simulink model "Defrost_3"  (R2022b)
settings: Solver=VariableStepAuto  StartTime=0.0  StopTime=100.0  RelTol=1e-3
InitFcn:
  | SNA = 170.5;
  | Temp_am = 4.5;
  | Tdef = 10;
  | Tdef_Second = 5;
  | Tbatt1 = 1;
  | Tbatt2 = 1;
  | RearDef_Voltage_L = 11.5;
  | RearDef_Voltage_H = 12;
undefined symbols (not defined in the file): sigbuilder_block
libraries: simulink x8
settings Model: Creator=muham  LastModifiedBy=muham

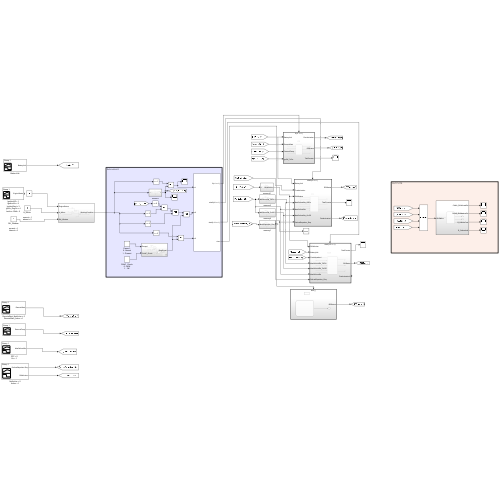
[thumbnail: Simulink's stored preview of the top-level diagram]
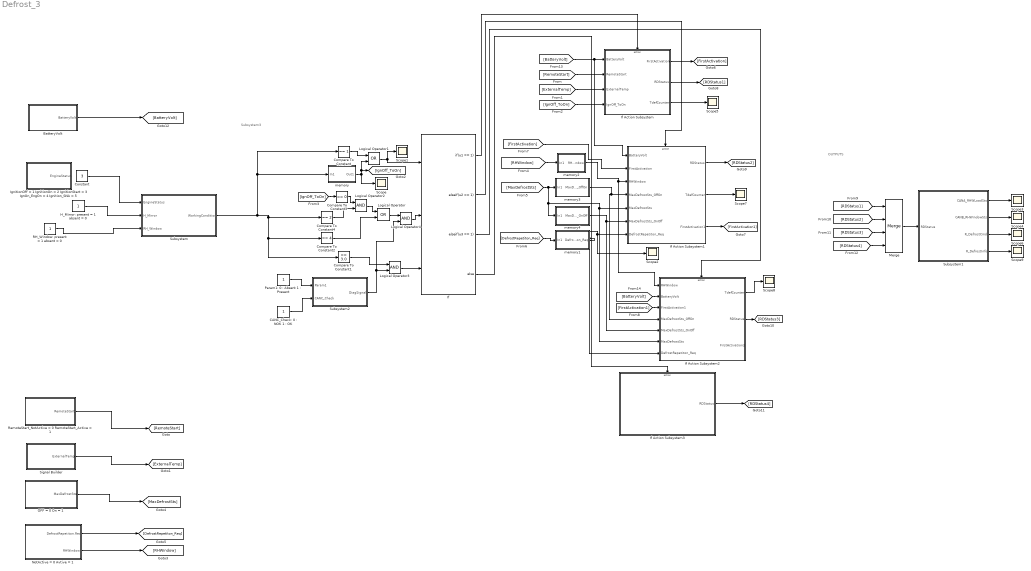
== system Defrost_3 ==
  note: Subsystem3
  note: OUTPUTS
  BatteryVolt : Subsystem  Tag=STV Subsys  LoadFcn=sigbuilder_block('load');  StartFcn=sigbuilder_block('start');  StopFcn=sigbuilder_block('stop');  ClipboardFcn=sigbuilder_block('clipboard');  mask(Sigbuilder block){tuvar=[0:10]}
      mask help: Simulink:masks:SigbuilderBlock_MD
      mask init:
      | if ~strcmp(get_param(bdroot(gcbh),'SimulationStatus'),'stopped') tuvar = sigbuilder_block('maskInit'); end
      settings: CopyFcn=sigbuilder_block('copy');  DeleteFcn=sigbuilder_block('delete');  ModelCloseFcn=sigbuilder_block('modelClose');  PreSaveFcn=sigbuilder_block('preSave');  PauseFcn=sigbuilder_block('pause');  ContinueFcn=sigbuilder_block('continue');  NameChangeFcn=sigbuilder_block('namechange');  OpenFcn=sigbuilder_block('open',[404.625 118.125 550.5 364.5 ]);  CloseFcn=sigbuilder_block('close');
      mask Display: plot(0, 0, 100, 100,[2, 2, 32, 32, 2], [68, 8, 8, 68, 68],[32, 2], [38, 38], [32, 19, 2],[53, 60, 44], [32, 17, 17, 2],[16, 16, 31, 31]);txt = getActiveGroup(gcbh);text(2, 100, txt,'verticalAlignment', 'top');
  "CANC_Check: 0 : NOK 1 : OK" : Constant
  Compare To Constant : simulink/Logic and Bit Operations/Compare To Constant  relop===  const=1  OutDataTypeStr=boolean
  Compare To Constant1 : simulink/Logic and Bit Operations/Compare To Constant  relop===  const=3.0  OutDataTypeStr=boolean
  Compare To Constant2 : simulink/Logic and Bit Operations/Compare To Constant  relop===  const=4  OutDataTypeStr=boolean
  Compare To Constant3 : simulink/Logic and Bit Operations/Compare To Constant  relop===  const=0  OutDataTypeStr=boolean
  Compare To Constant4 : simulink/Logic and Bit Operations/Compare To Constant  relop===  const=2  OutDataTypeStr=boolean
  Constant : Constant  Value=3
  H_Mirror: present = 1 absent = 0 : Constant
  If : If  NumInputs=3  IfExpression=u1 == 1  ElseIfExpressions=u2 == 1, u3 == 1
  If Action Subsystem : Subsystem  TreatAsAtomicUnit=on
  If Action Subsystem1 : Subsystem  TreatAsAtomicUnit=on
  If Action Subsystem2 : Subsystem  TreatAsAtomicUnit=on
  If Action Subsystem3 : Subsystem  TreatAsAtomicUnit=on
  IgnitionOff = 1 IgnitionOn = 2 IgnitionStart = 3 IgnOn_EngOn = 4 Ignition_SNA = 5 : Subsystem  Tag=STV Subsys  LoadFcn=sigbuilder_block('load');  StartFcn=sigbuilder_block('start');  StopFcn=sigbuilder_block('stop');  ClipboardFcn=sigbuilder_block('clipboard');  mask(Sigbuilder block){tuvar=[0:10]}
      mask help: Simulink:masks:SigbuilderBlock_MD
      mask init:
      | if ~strcmp(get_param(bdroot(gcbh),'SimulationStatus'),'stopped') tuvar = sigbuilder_block('maskInit'); end
      settings: CopyFcn=sigbuilder_block('copy');  DeleteFcn=sigbuilder_block('delete');  ModelCloseFcn=sigbuilder_block('modelClose');  PreSaveFcn=sigbuilder_block('preSave');  PauseFcn=sigbuilder_block('pause');  ContinueFcn=sigbuilder_block('continue');  NameChangeFcn=sigbuilder_block('namechange');  OpenFcn=sigbuilder_block('open',[73.125 79.125 550.5 364.5 ]);  CloseFcn=sigbuilder_block('close');
      mask Display: plot(0, 0, 100, 100,[2, 2, 32, 32, 2], [68, 8, 8, 68, 68],[32, 2], [38, 38], [32, 19, 2],[53, 60, 44], [32, 17, 17, 2],[16, 16, 31, 31]);txt = getActiveGroup(gcbh);text(2, 100, txt,'verticalAlignment', 'top');
  Logical Operator : Logic  Operator=OR  AllPortsSameDT=off  OutDataTypeStr=boolean
  Logical Operator1 : Logic  Operator=OR  AllPortsSameDT=off  OutDataTypeStr=boolean
  Logical Operator2 : Logic  AllPortsSameDT=off  OutDataTypeStr=boolean
  Logical Operator3 : Logic  AllPortsSameDT=off  OutDataTypeStr=boolean
  Logical Operator4 : Logic  AllPortsSameDT=off  OutDataTypeStr=boolean
  Merge : Merge  Inputs=4
  NotActive = 0 Avtive = 1 : Subsystem  Tag=STV Subsys  LoadFcn=sigbuilder_block('load');  StartFcn=sigbuilder_block('start');  StopFcn=sigbuilder_block('stop');  ClipboardFcn=sigbuilder_block('clipboard');  mask(Sigbuilder block){tuvar=[0:10]}
      mask help: Simulink:masks:SigbuilderBlock_MD
      mask init:
      | if ~strcmp(get_param(bdroot(gcbh),'SimulationStatus'),'stopped') tuvar = sigbuilder_block('maskInit'); end
      settings: CopyFcn=sigbuilder_block('copy');  DeleteFcn=sigbuilder_block('delete');  ModelCloseFcn=sigbuilder_block('modelClose');  PreSaveFcn=sigbuilder_block('preSave');  PauseFcn=sigbuilder_block('pause');  ContinueFcn=sigbuilder_block('continue');  NameChangeFcn=sigbuilder_block('namechange');  OpenFcn=sigbuilder_block('open',[404.625 118.125 550.5 364.5 ]);  CloseFcn=sigbuilder_block('close');
      mask Display: plot(0, 0, 100, 100,[2, 2, 32, 32, 2], [68, 8, 8, 68, 68],[32, 2], [38, 38], [32, 19, 2],[53, 60, 44], [32, 17, 17, 2],[16, 16, 31, 31]);txt = getActiveGroup(gcbh);text(2, 100, txt,'verticalAlignment', 'top');
  OFF = 0 On = 1 : Subsystem  Tag=STV Subsys  LoadFcn=sigbuilder_block('load');  StartFcn=sigbuilder_block('start');  StopFcn=sigbuilder_block('stop');  ClipboardFcn=sigbuilder_block('clipboard');  mask(Sigbuilder block){tuvar=[0:10]}
      mask help: Simulink:masks:SigbuilderBlock_MD
      mask init:
      | if ~strcmp(get_param(bdroot(gcbh),'SimulationStatus'),'stopped') tuvar = sigbuilder_block('maskInit'); end
      settings: CopyFcn=sigbuilder_block('copy');  DeleteFcn=sigbuilder_block('delete');  ModelCloseFcn=sigbuilder_block('modelClose');  PreSaveFcn=sigbuilder_block('preSave');  PauseFcn=sigbuilder_block('pause');  ContinueFcn=sigbuilder_block('continue');  NameChangeFcn=sigbuilder_block('namechange');  OpenFcn=sigbuilder_block('open',[404.625 118.125 550.5 364.5 ]);  CloseFcn=sigbuilder_block('close');
      mask Display: plot(0, 0, 100, 100,[2, 2, 32, 32, 2], [68, 8, 8, 68, 68],[32, 2], [38, 38], [32, 19, 2],[53, 60, 44], [32, 17, 17, 2],[16, 16, 31, 31]);txt = getActiveGroup(gcbh);text(2, 100, txt,'verticalAlignment', 'top');
  "Param1: 0 : Absent 1 : Present" : Constant
  RH_Window: present = 1 absent = 0 : Constant
  RemoteStart_NotActive = 0 RemoteStart_Active = 1 : Subsystem  Tag=STV Subsys  LoadFcn=sigbuilder_block('load');  StartFcn=sigbuilder_block('start');  StopFcn=sigbuilder_block('stop');  ClipboardFcn=sigbuilder_block('clipboard');  mask(Sigbuilder block){tuvar=[0:10]}
      mask help: Simulink:masks:SigbuilderBlock_MD
      mask init:
      | if ~strcmp(get_param(bdroot(gcbh),'SimulationStatus'),'stopped') tuvar = sigbuilder_block('maskInit'); end
      settings: CopyFcn=sigbuilder_block('copy');  DeleteFcn=sigbuilder_block('delete');  ModelCloseFcn=sigbuilder_block('modelClose');  PreSaveFcn=sigbuilder_block('preSave');  PauseFcn=sigbuilder_block('pause');  ContinueFcn=sigbuilder_block('continue');  NameChangeFcn=sigbuilder_block('namechange');  OpenFcn=sigbuilder_block('open',[404.625 118.125 550.5 364.5 ]);  CloseFcn=sigbuilder_block('close');
      mask Display: plot(0, 0, 100, 100,[2, 2, 32, 32, 2], [68, 8, 8, 68, 68],[32, 2], [38, 38], [32, 19, 2],[53, 60, 44], [32, 17, 17, 2],[16, 16, 31, 31]);txt = getActiveGroup(gcbh);text(2, 100, txt,'verticalAlignment', 'top');
  Scope{,1..9} (10 alike) : Scope
  Signal Builder : Subsystem  Tag=STV Subsys  LoadFcn=sigbuilder_block('load');  StartFcn=sigbuilder_block('start');  StopFcn=sigbuilder_block('stop');  ClipboardFcn=sigbuilder_block('clipboard');  mask(Sigbuilder block){tuvar=[0:10]}
      mask help: Simulink:masks:SigbuilderBlock_MD
      mask init:
      | if ~strcmp(get_param(bdroot(gcbh),'SimulationStatus'),'stopped') tuvar = sigbuilder_block('maskInit'); end
      settings: CopyFcn=sigbuilder_block('copy');  DeleteFcn=sigbuilder_block('delete');  ModelCloseFcn=sigbuilder_block('modelClose');  PreSaveFcn=sigbuilder_block('preSave');  PauseFcn=sigbuilder_block('pause');  ContinueFcn=sigbuilder_block('continue');  NameChangeFcn=sigbuilder_block('namechange');  OpenFcn=sigbuilder_block('open',[404.625 118.125 550.5 364.5 ]);  CloseFcn=sigbuilder_block('close');
      mask Display: plot(0, 0, 100, 100,[2, 2, 32, 32, 2], [68, 8, 8, 68, 68],[32, 2], [38, 38], [32, 19, 2],[53, 60, 44], [32, 17, 17, 2],[16, 16, 31, 31]);txt = getActiveGroup(gcbh);text(2, 100, txt,'verticalAlignment', 'top');
  Subsystem : Subsystem
  Subsystem1 : Subsystem
  Subsystem2 : Subsystem
  memory : Subsystem
  memory1 : Subsystem
  memory2 : Subsystem
  memory3 : Subsystem
  memory4 : Subsystem
  wires:
  Signal Builder/1(ExternalTemp) -> [ExternalTemp]
  RemoteStart_NotActive = 0 RemoteStart_Active = 1/1(RemoteStart) -> [RemoteStart]
  [IgnOff_ToOn] -> If Action Subsystem/4(IgnOff_ToOn)
  [RemoteStart] -> If Action Subsystem/2(RemoteStart)
  [ExternalTemp] -> If Action Subsystem/3(ExternalTemp)
  [DefrostRepetiton_Req] -> memory1/1(In1)
  memory3/1(MaxDefrostSts_OffOn) -> If Action Subsystem2/4(MaxDefrostSts_OffOn), If Action Subsystem1/4(MaxDefrostSts_OffOn)
  memory2/1(RHWindow) -> If Action Subsystem1/3(RHWindow), If Action Subsystem2/1(RHWindow)
  [RHWindow] -> memory2/1(In1)
  NotActive = 0 Avtive = 1/1(DefrostRepetiton.Req) -> [DefrostRepetiton_Req]
  memory1/1(DefrostRepetiton_Req) -> If Action Subsystem1/7(DefrostRepetiton_Req), Scope2/1, If Action Subsystem2/7(DefrostRepetiton_Req)
  NotActive = 0 Avtive = 1/2(RHWindow) -> [RHWindow]
  OFF = 0 On = 1/1(MaxDefrostSts) -> [MaxDefrostSts]
  If Action Subsystem/1(FirstActivation) -> [FirstActivation]
  If Action Subsystem/2(RDStatus) -> [RDStatus1]
  If Action Subsystem/3(TdefCounter) -> Scope5/1
  If Action Subsystem1/1(RDStatus) -> [RDStatus2]
  If Action Subsystem1/2(TdefCounter) -> Scope7/1
  If Action Subsystem2/1(TdefCounter) -> Scope8/1
  If Action Subsystem2/2(RDStatus) -> [RDStatus3]
  memory4/1(MaxDefrostSts_OnOff) -> If Action Subsystem1/6(MaxDefrostSts_OnOff), If Action Subsystem2/5(MaxDefrostSts_OnOff)
  If Action Subsystem1/3(FirstActivation1) -> [FirstActivation1]
  [MaxDefrostSts] -> memory4/1(In1), If Action Subsystem2/6(MaxDefrostSts), If Action Subsystem1/5(MaxDefrostSts), memory3/1(In1)
  [FirstActivation] -> If Action Subsystem1/2(FirstActivation)
  [FirstActivation1] -> If Action Subsystem2/3(FirstActivation1)
  If Action Subsystem3/1(RDStatus) -> [RDStatus4]
  [RDStatus1] -> Merge/1
  [RDStatus2] -> Merge/2
  [RDStatus3] -> Merge/3
  [RDStatus4] -> Merge/4
  BatteryVolt/1(BatteryVolt) -> [BatteryVolt]
  [BatteryVolt] -> If Action Subsystem1/1(BatteryVolt), If Action Subsystem/1(BatteryVolt)
  [BatteryVolt] -> If Action Subsystem2/2(BatteryVolt)
  Constant/1 -> Subsystem/1(EngineStatus)
  Merge/1 -> Subsystem1/1(RDStatus)
  Subsystem1/1(CANA_RHWLoadSts) -> Scope3/1
  Subsystem1/2(CANB_RHWindowSts) -> Scope4/1
  Subsystem1/3(R_DefrostCmd) -> Scope6/1
  Subsystem1/4(R_DefrostInfo) -> Scope9/1
  H_Mirror: present = 1 absent = 0/1 -> Subsystem/2(H_Mirror)
  RH_Window: present = 1 absent = 0/1 -> Subsystem/3(RH_Window)
  If/1 -> If Action Subsystem/Action
  If/2 -> If Action Subsystem1/Action
  If/3 -> If Action Subsystem2/Action
  If/4 -> If Action Subsystem3/Action
  "Param1: 0 : Absent 1 : Present"/1 -> Subsystem2/1(Param1)
  Logical Operator/1 -> Logical Operator4/1
  Compare To Constant3/1 -> Logical Operator2/1
  "CANC_Check: 0 : NOK 1 : OK"/1 -> Subsystem2/2(CANC_Check)
  Compare To Constant4/1 -> Logical Operator2/2
  Logical Operator2/1 -> Logical Operator/1
  Compare To Constant2/1 -> Logical Operator/2
  Compare To Constant/1 -> Logical Operator1/1
  Logical Operator4/1 -> If/2
  Subsystem/1(WorkingCondition) -> Compare To Constant1/1, Compare To Constant2/1, Compare To Constant4/1, Compare To Constant/1, memory/1(In1)
  Compare To Constant1/1 -> Logical Operator3/1
  Subsystem2/1(DiagSignal) -> Logical Operator4/2, Logical Operator3/2
  Logical Operator3/1 -> If/3
  memory/1(Out1) -> Scope/1, Logical Operator1/2, [IgnOff_ToOn]
  [IgnOff_ToOn] -> Compare To Constant3/1
  Logical Operator1/1 -> Scope1/1, If/1

== system Defrost_3/BatteryVolt ==
  Demux : Demux  Tag=STV Demux  Outputs=1
      settings: DisplayOption=none
  FromWs : FromWorkspace  Tag=STV FromWs  VariableName=tuvar
      SigBuilderData=|
      | common.afterFinalStr = 'Extrapolate'
      | common.sampleTime = 0
      | dataSet.timeRange = [0 100]
      | dataSet.name = 'Group 1'
      | sbobj.Groups.Name = 'Group 1'
      | sbobj.Groups.Signals.Name = 'BatteryVolt'
      | sbobj.Groups.Signals.XData = [0 8.33333333333 8.33333333333 16.6666666667 25 25 33.3333333333 33.3333333333 41.6666666667 41.6666666667 50 50 58.3333333333 58.3333333333 66.6666666667 66.6666666667 75 75 83.3333333333 83.3333333333 91.6666666667 91.6666666667 100]
      | sbobj.Groups.Signals.YData = [2 2 3.98 3.98 3.98 6.78 6.78 7.05 7.05 11.85 11.85 24.3 24.3 31.2 31.2 36.2 36.2 21 21 11.2 11.2 4.8 4.8]
      | sbobj.Groups.TimeRange = [0 100]
  BatteryVolt : Outport  Tag=STV Outport
  wires:
  Demux/1 -> BatteryVolt/1
  FromWs/1 -> Demux/1

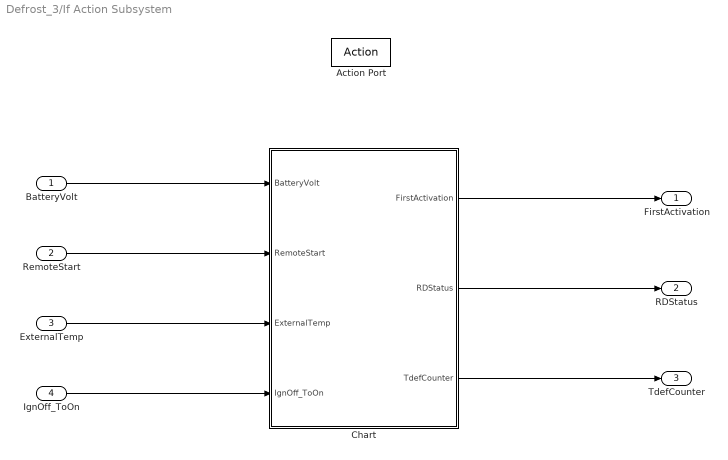
== system Defrost_3/If Action Subsystem ==
  BatteryVolt : Inport
  RemoteStart : Inport  Port=2
  ExternalTemp : Inport  Port=3
  IgnOff_ToOn : Inport  Port=4
  Action Port : ActionPort  ActionPortLabel=if(u1 == 1)
  Chart : Stateflow chart  TreatAsAtomicUnit=on
  FirstActivation : Outport
  RDStatus : Outport  Port=2
  TdefCounter : Outport  Port=3
  wires:
  ExternalTemp/1 -> Chart/3(ExternalTemp)
  IgnOff_ToOn/1 -> Chart/4(IgnOff_ToOn)
  Chart/1(FirstActivation) -> FirstActivation/1
  Chart/2(RDStatus) -> RDStatus/1
  Chart/3(TdefCounter) -> TdefCounter/1
  RemoteStart/1 -> Chart/2(RemoteStart)
  BatteryVolt/1 -> Chart/1(BatteryVolt)

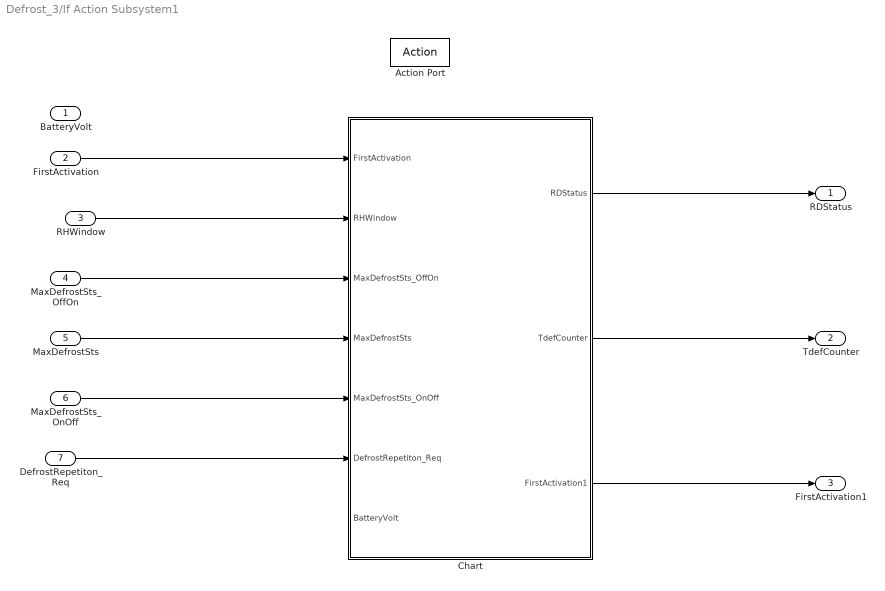
== system Defrost_3/If Action Subsystem1 ==
  BatteryVolt : Inport
  FirstActivation : Inport  Port=2
  RHWindow : Inport  Port=3
  MaxDefrostSts_OffOn : Inport  Port=4
  MaxDefrostSts : Inport  Port=5
  MaxDefrostSts_OnOff : Inport  Port=6
  DefrostRepetiton_Req : Inport  Port=7
  Action Port : ActionPort  ActionPortLabel=elseif(u2 == 1)
  Chart : Stateflow chart  TreatAsAtomicUnit=on
  RDStatus : Outport
  TdefCounter : Outport  Port=2
  FirstActivation1 : Outport  Port=3
  wires:
  MaxDefrostSts_OffOn/1 -> Chart/3(MaxDefrostSts_OffOn)
  DefrostRepetiton_Req/1 -> Chart/6(DefrostRepetiton_Req)
  RHWindow/1 -> Chart/2(RHWindow)
  Chart/2(TdefCounter) -> TdefCounter/1
  Chart/1(RDStatus) -> RDStatus/1
  MaxDefrostSts/1 -> Chart/4(MaxDefrostSts)
  FirstActivation/1 -> Chart/1(FirstActivation)
  MaxDefrostSts_OnOff/1 -> Chart/5(MaxDefrostSts_OnOff)
  Chart/3(FirstActivation1) -> FirstActivation1/1

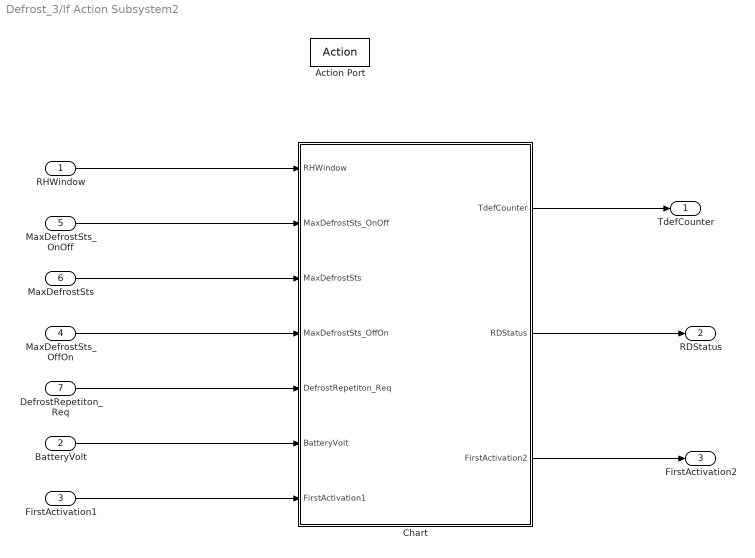
== system Defrost_3/If Action Subsystem2 ==
  RHWindow : Inport
  BatteryVolt : Inport  Port=2
  FirstActivation1 : Inport  Port=3
  MaxDefrostSts_OffOn : Inport  Port=4
  MaxDefrostSts_OnOff : Inport  Port=5
  MaxDefrostSts : Inport  Port=6
  DefrostRepetiton_Req : Inport  Port=7
  Action Port : ActionPort  ActionPortLabel=elseif( u3 == 1)
  Chart : Stateflow chart  TreatAsAtomicUnit=on
      settings: PortSchema="{\"entries\":[{\"content\":{\"sides\":[{\"content\":{\"connectorIds\":[\"In2\",\"In3\",\"In4\",\"In5\",\"In6\",\"In7\",\"In1\"]},\"type\":\"ConnectorPlacement.EquallySpacedRectSide\",\"uuid\":\"5c558dba-9868-4eda-8643-b95f5a3e8853\"},{\"content\":{\"connectorIds\":[\"Out1\",\"Out2\",\"Out3\"],\"side\":\"RIGHT\"},\"type\":\"ConnectorPlacement.EquallySpacedRectSide\",\"uuid\":\"4f0894d4-817e-4352-92d3-82fb3ad90bd1\"},{\"content\":{\"connectorIds\":[],\"side\":\"TOP\"},\"type\":\"ConnectorPlacement.EquallySpacedRectSide\",\"uuid\":\"ff8b1fba-ba2b-4d5b-bd2f-e45e2071cdfd\"},{\"content\":{\"connectorIds\":[],\"side\":\"BOTTOM\"},\"type\":\"ConnectorPlacement.EquallySpacedRectSide\",\"uuid\":\"6154f71e-1b79-4ae1-a680-58474921fd4e\"}]},\"type\":\"ConnectorPlacement.EquallySpacedConnector\",\"uuid\":\"73fac0a1-d9ca-445b-bae0-3ca66b8dc5da\"}],\"packageUris\":[\"http://schema.mathworks.com/mf0/Connector/R2020b\"],\"version\":\"1.0\"}"
  TdefCounter : Outport
  RDStatus : Outport  Port=2
  FirstActivation2 : Outport  Port=3
  wires:
  RHWindow/1 -> Chart/2(RHWindow)
  MaxDefrostSts/1 -> Chart/4(MaxDefrostSts)
  DefrostRepetiton_Req/1 -> Chart/6(DefrostRepetiton_Req)
  Chart/1(TdefCounter) -> TdefCounter/1
  Chart/2(RDStatus) -> RDStatus/1
  MaxDefrostSts_OnOff/1 -> Chart/3(MaxDefrostSts_OnOff)
  MaxDefrostSts_OffOn/1 -> Chart/5(MaxDefrostSts_OffOn)
  FirstActivation1/1 -> Chart/1(FirstActivation1)
  Chart/3(FirstActivation2) -> FirstActivation2/1
  BatteryVolt/1 -> Chart/7(BatteryVolt)

== system Defrost_3/If Action Subsystem3 ==
  Action Port : ActionPort  ActionPortLabel=else
  Chart : Stateflow chart  TreatAsAtomicUnit=on
  RDStatus : Outport
  wires:
  Chart/1(RDStatus) -> RDStatus/1

== system Defrost_3/IgnitionOff = 1 IgnitionOn = 2 IgnitionStart = 3 IgnOn_EngOn = 4 Ignition_SNA = 5 ==
  Demux : Demux  Tag=STV Demux  Outputs=1
      settings: DisplayOption=none
  FromWs : FromWorkspace  Tag=STV FromWs  VariableName=tuvar
      SigBuilderData=|
      | common.afterFinalStr = 'Extrapolate'
      | common.sampleTime = 0
      | dataSet.timeRange = [0 100]
      | dataSet.name = 'Group 1'
      | sbobj.Groups.Name = 'Group 1'
      | sbobj.Groups.Signals.Name = 'EngineStatus'
      | sbobj.Groups.Signals.XData = [0 5 5 10 10 15 15 20 20 25 25 30 30 35 35 40 40 45 45 50 50 55 55 60 60 65 65 70 70 75 75 80 80 85 85 90 90 95 95 100]
      | sbobj.Groups.Signals.YData = [1 1 2 2 3 3 4 4 3 3 2 2 1 1 2 2 3 3 4 4 3 3 2 2 1 1 2 2 3 3 4 4 3 3 2 2 1 1 2 2]
      | sbobj.Groups.TimeRange = [0 100]
  EngineStatus : Outport  Tag=STV Outport
  wires:
  Demux/1 -> EngineStatus/1
  FromWs/1 -> Demux/1

== system Defrost_3/NotActive = 0 Avtive = 1 ==
  Demux : Demux  Tag=STV Demux  Outputs=2
      settings: DisplayOption=none
  FromWs : FromWorkspace  Tag=STV FromWs  VariableName=tuvar
      SigBuilderData=|
      | common.afterFinalStr = 'Extrapolate'
      | common.sampleTime = 0
      | dataSet.timeRange = [0 100]
      | dataSet.name = 'Group 1'
      | sbobj.Groups.Name = 'Group 1'
      | sbobj.Groups.Signals(1).Name = 'DefrostRepetiton.Req'
      | sbobj.Groups.Signals(1).XData = [0 5 10 10 15 15 20 20 25 25 30 30 35 35 40 40 45 45 50 50 55 55 60 60 65 65 70 70 75 75 80 80 85 85 90 90 95 95 100]
      | sbobj.Groups.Signals(1).YData = [0 0 0 1 1 0 0 1 1 0 0 1 1 0 0 1 1 0 0 1 1 0 0 1 1 0 0 1 1 0 0 1 1 0 0 1 1 0 0]
      | sbobj.Groups.Signals(2).Name = 'RHWindow'
      | sbobj.Groups.Signals(2).XData = [0 5 10 15 15 20 25 30 30 35 40 45 45 50 55 60 60 65 70 75 75 80 85 90 90 95 100]
      | sbobj.Groups.Signals(2).YData = [1 1 1 1 0 0 0 0 1 1 1 1 0 0 0 0 1 1 1 1 0 0 0 0 1 1 1]
      | sbobj.Groups.TimeRange = [0 100]
  DefrostRepetiton.Req : Outport  Tag=STV Outport
  RHWindow : Outport  Tag=STV Outport  Port=2
  wires:
  Demux/1 -> DefrostRepetiton.Req/1
  FromWs/1 -> Demux/1
  Demux/2 -> RHWindow/1

== system Defrost_3/OFF = 0 On = 1 ==
  Demux : Demux  Tag=STV Demux  Outputs=1
      settings: DisplayOption=none
  FromWs : FromWorkspace  Tag=STV FromWs  VariableName=tuvar
      SigBuilderData=|
      | common.afterFinalStr = 'Extrapolate'
      | common.sampleTime = 0
      | dataSet.timeRange = [0 100]
      | dataSet.name = 'Group 1'
      | sbobj.Groups.Name = 'Group 1'
      | sbobj.Groups.Signals.Name = 'MaxDefrostSts'
      | sbobj.Groups.Signals.XData = [0 5 10 10 15 20 20 25 30 30 35 40 40 45 50 50 55 60 60 65 70 70 75 80 80 85 90 90 95 100]
      | sbobj.Groups.Signals.YData = [1 1 1 0 0 0 1 1 1 0 0 0 1 1 1 0 0 0 1 1 1 0 0 0 1 1 1 0 0 0]
      | sbobj.Groups.TimeRange = [0 100]
  MaxDefrostSts : Outport  Tag=STV Outport
  wires:
  Demux/1 -> MaxDefrostSts/1
  FromWs/1 -> Demux/1

== system Defrost_3/RemoteStart_NotActive = 0 RemoteStart_Active = 1 ==
  Demux : Demux  Tag=STV Demux  Outputs=1
      settings: DisplayOption=none
  FromWs : FromWorkspace  Tag=STV FromWs  VariableName=tuvar
      SigBuilderData=|
      | common.afterFinalStr = 'Extrapolate'
      | common.sampleTime = 0
      | dataSet.timeRange = [0 100]
      | dataSet.name = 'Group 1'
      | sbobj.Groups.Name = 'Group 1'
      | sbobj.Groups.Signals.Name = 'RemoteStart'
      | sbobj.Groups.Signals.XData = [0 5 5 10 15 20 20 25 30 30 35 40 40 45 50 50 55 60 60 65 70 70 75 80 80 85 90 95 95 100]
      | sbobj.Groups.Signals.YData = [1 1 0 0 0 0 1 1 1 0 0 0 1 1 1 0 0 0 1 1 1 0 0 0 1 1 1 1 0 0]
      | sbobj.Groups.TimeRange = [0 100]
  RemoteStart : Outport  Tag=STV Outport
  wires:
  Demux/1 -> RemoteStart/1
  FromWs/1 -> Demux/1

== system Defrost_3/Signal Builder ==
  Demux : Demux  Tag=STV Demux  Outputs=1
      settings: DisplayOption=none
  FromWs : FromWorkspace  Tag=STV FromWs  VariableName=tuvar
      SigBuilderData=|
      | common.afterFinalStr = 'Extrapolate'
      | common.sampleTime = 0
      | dataSet.timeRange = [0 100]
      | dataSet.name = 'Group 1'
      | sbobj.Groups.Name = 'Group 1'
      | sbobj.Groups.Signals.Name = 'ExternalTemp'
      | sbobj.Groups.Signals.XData = [0 5 10 15 15 20 25 25 30 35 35 40 40 45 50 50 55 55 60 60 65 65 70 70 75 80 85 85 90 90 95 95 100]
      | sbobj.Groups.Signals.YData = [-26 -26 -26 -26 -3 -3 -3 2.05 2.05 2.05 2 2 2.05 2.05 2.05 170.5 170.5 171 171 172 172 180 180 177 177 177 177 180 180 178 178 176 176]
      | sbobj.Groups.TimeRange = [0 100]
  ExternalTemp : Outport  Tag=STV Outport
  wires:
  Demux/1 -> ExternalTemp/1
  FromWs/1 -> Demux/1

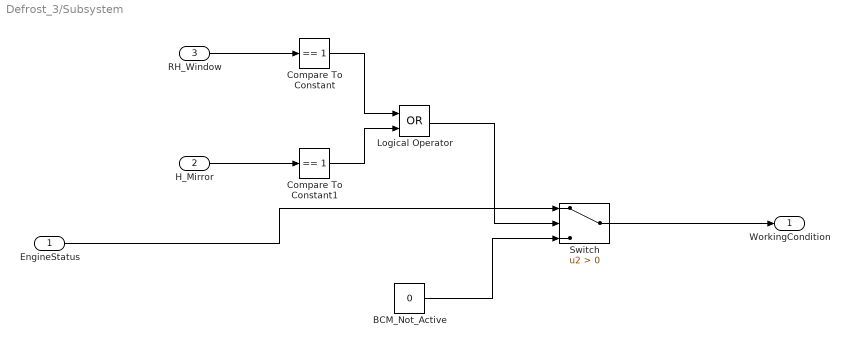
== system Defrost_3/Subsystem ==
  EngineStatus : Inport
  H_Mirror : Inport  Port=2
  RH_Window : Inport  Port=3
  BCM_Not_Active : Constant  Value=0
  Compare To Constant : simulink/Logic and Bit Operations/Compare To Constant  relop===  const=1  OutDataTypeStr=boolean
  Compare To Constant1 : simulink/Logic and Bit Operations/Compare To Constant  relop===  const=1  OutDataTypeStr=boolean
  Logical Operator : Logic  Operator=OR  AllPortsSameDT=off  OutDataTypeStr=boolean
  Switch : Switch  Criteria=u2 > Threshold  SaturateOnIntegerOverflow=off  InputSameDT=off
  WorkingCondition : Outport
  wires:
  H_Mirror/1 -> Compare To Constant1/1
  RH_Window/1 -> Compare To Constant/1
  Compare To Constant/1 -> Logical Operator/1
  Compare To Constant1/1 -> Logical Operator/2
  Logical Operator/1 -> Switch/2
  EngineStatus/1 -> Switch/1
  BCM_Not_Active/1 -> Switch/3
  Switch/1 -> WorkingCondition/1

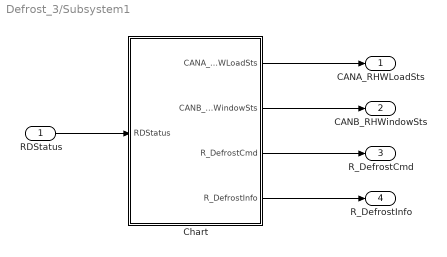
== system Defrost_3/Subsystem1 ==
  RDStatus : Inport
  Chart : Stateflow chart  TreatAsAtomicUnit=on
  CANA_RHWLoadSts : Outport
  CANB_RHWindowSts : Outport  Port=2
  R_DefrostCmd : Outport  Port=3
  R_DefrostInfo : Outport  Port=4
  wires:
  Chart/2(CANB_RHWindowSts) -> CANB_RHWindowSts/1
  Chart/1(CANA_RHWLoadSts) -> CANA_RHWLoadSts/1
  RDStatus/1 -> Chart/1(RDStatus)
  Chart/4(R_DefrostInfo) -> R_DefrostInfo/1
  Chart/3(R_DefrostCmd) -> R_DefrostCmd/1

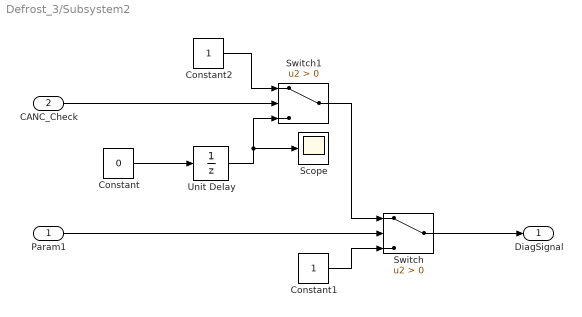
== system Defrost_3/Subsystem2 ==
  Param1 : Inport
  CANC_Check : Inport  Port=2
  Constant : Constant  Value=0
  Constant1 : Constant
  Constant2 : Constant
  Scope : Scope
  Switch : Switch  Criteria=u2 > Threshold  SaturateOnIntegerOverflow=off  InputSameDT=off
  Switch1 : Switch  Criteria=u2 > Threshold  SaturateOnIntegerOverflow=off  InputSameDT=off
  Unit Delay : UnitDelay  InitialCondition=1  SampleTime=0.0025  HasFrameUpgradeWarning=on
  DiagSignal : Outport
  wires:
  Param1/1 -> Switch/2
  Constant1/1 -> Switch/3
  CANC_Check/1 -> Switch1/2
  Switch1/1 -> Switch/1
  Constant2/1 -> Switch1/1
  Constant/1 -> Unit Delay/1
  Unit Delay/1 -> Scope/1, Switch1/3
  Switch/1 -> DiagSignal/1

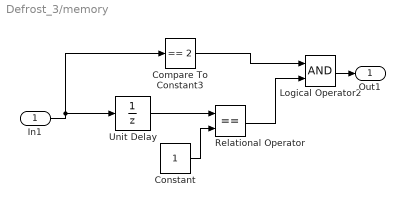
== system Defrost_3/memory ==
  In1 : Inport
  Compare To Constant3 : simulink/Logic and Bit Operations/Compare To Constant  relop===  const=2  OutDataTypeStr=boolean
  Constant : Constant
  Logical Operator2 : Logic  AllPortsSameDT=off  OutDataTypeStr=boolean
  Relational Operator : RelationalOperator  Operator===  OutDataTypeStr=boolean  RndMeth=Simplest  InputSameDT=off
  Unit Delay : UnitDelay  SampleTime=5  HasFrameUpgradeWarning=on
  Out1 : Outport
  wires:
  Constant/1 -> Relational Operator/2
  Unit Delay/1 -> Relational Operator/1
  Logical Operator2/1 -> Out1/1
  Relational Operator/1 -> Logical Operator2/2
  In1/1 -> Compare To Constant3/1, Unit Delay/1
  Compare To Constant3/1 -> Logical Operator2/1

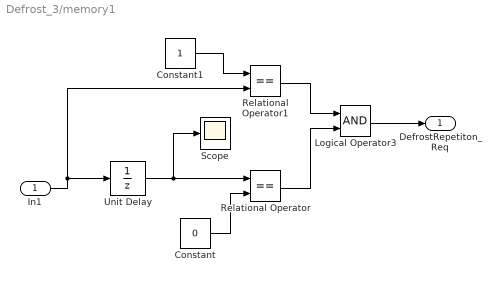
== system Defrost_3/memory1 ==
  In1 : Inport
  Constant : Constant  Value=0
  Constant1 : Constant
  Logical Operator3 : Logic  AllPortsSameDT=off  OutDataTypeStr=boolean
  Relational Operator : RelationalOperator  Operator===  OutDataTypeStr=boolean  RndMeth=Simplest  InputSameDT=off
  Relational Operator1 : RelationalOperator  Operator===  OutDataTypeStr=boolean  RndMeth=Simplest  InputSameDT=off
  Scope : Scope
  Unit Delay : UnitDelay  SampleTime=5  HasFrameUpgradeWarning=on
  DefrostRepetiton_Req : Outport
  wires:
  In1/1 -> Unit Delay/1, Relational Operator1/2
  Unit Delay/1 -> Scope/1, Relational Operator/1
  Constant/1 -> Relational Operator/2
  Relational Operator1/1 -> Logical Operator3/1
  Constant1/1 -> Relational Operator1/1
  Relational Operator/1 -> Logical Operator3/2
  Logical Operator3/1 -> DefrostRepetiton_Req/1

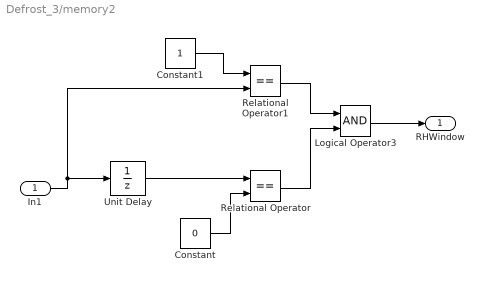
== system Defrost_3/memory2 ==
  In1 : Inport
  Constant : Constant  Value=0
  Constant1 : Constant
  Logical Operator3 : Logic  AllPortsSameDT=off  OutDataTypeStr=boolean
  Relational Operator : RelationalOperator  Operator===  OutDataTypeStr=boolean  RndMeth=Simplest  InputSameDT=off
  Relational Operator1 : RelationalOperator  Operator===  OutDataTypeStr=boolean  RndMeth=Simplest  InputSameDT=off
  Unit Delay : UnitDelay  SampleTime=5  HasFrameUpgradeWarning=on
  RHWindow : Outport
  wires:
  Logical Operator3/1 -> RHWindow/1
  Relational Operator/1 -> Logical Operator3/2
  Constant1/1 -> Relational Operator1/1
  Relational Operator1/1 -> Logical Operator3/1
  Constant/1 -> Relational Operator/2
  Unit Delay/1 -> Relational Operator/1
  In1/1 -> Relational Operator1/2, Unit Delay/1

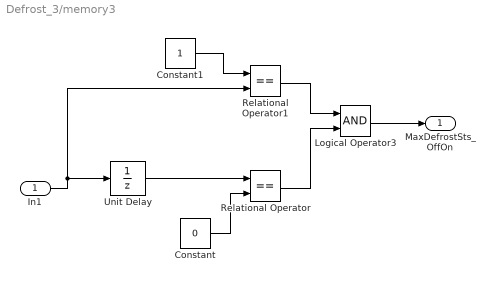
== system Defrost_3/memory3 ==
  In1 : Inport
  Constant : Constant  Value=0
  Constant1 : Constant
  Logical Operator3 : Logic  AllPortsSameDT=off  OutDataTypeStr=boolean
  Relational Operator : RelationalOperator  Operator===  OutDataTypeStr=boolean  RndMeth=Simplest  InputSameDT=off
  Relational Operator1 : RelationalOperator  Operator===  OutDataTypeStr=boolean  RndMeth=Simplest  InputSameDT=off
  Unit Delay : UnitDelay  SampleTime=5  HasFrameUpgradeWarning=on
  MaxDefrostSts_OffOn : Outport
  wires:
  Logical Operator3/1 -> MaxDefrostSts_OffOn/1
  Relational Operator/1 -> Logical Operator3/2
  Constant1/1 -> Relational Operator1/1
  Relational Operator1/1 -> Logical Operator3/1
  Constant/1 -> Relational Operator/2
  Unit Delay/1 -> Relational Operator/1
  In1/1 -> Relational Operator1/2, Unit Delay/1

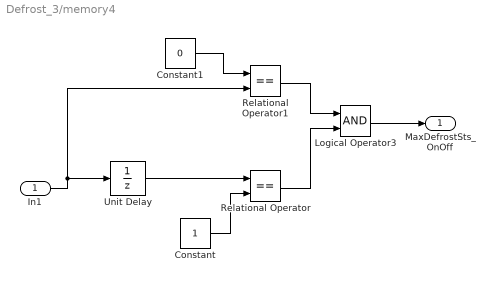
== system Defrost_3/memory4 ==
  In1 : Inport
  Constant : Constant
  Constant1 : Constant  Value=0
  Logical Operator3 : Logic  AllPortsSameDT=off  OutDataTypeStr=boolean
  Relational Operator : RelationalOperator  Operator===  OutDataTypeStr=boolean  RndMeth=Simplest  InputSameDT=off
  Relational Operator1 : RelationalOperator  Operator===  OutDataTypeStr=boolean  RndMeth=Simplest  InputSameDT=off
  Unit Delay : UnitDelay  SampleTime=5  HasFrameUpgradeWarning=on
  MaxDefrostSts_OnOff : Outport
  wires:
  In1/1 -> Unit Delay/1, Relational Operator1/2
  Unit Delay/1 -> Relational Operator/1
  Constant/1 -> Relational Operator/2
  Relational Operator1/1 -> Logical Operator3/1
  Constant1/1 -> Relational Operator1/1
  Relational Operator/1 -> Logical Operator3/2
  Logical Operator3/1 -> MaxDefrostSts_OnOff/1

== stateflow chart Defrost_3/If Action Subsystem2/Chart ==
  state Load_Shed_Management [parallel]
    settings: executionOrder=1
    state LowVoltage
    state Normal
    state HighVoltage
    (default) -> LowVoltage
    LowVoltage -> Normal : [BatteryVolt > RearDef_Voltage_L]
    Normal -> LowVoltage [order 1] : [BatteryVolt <= RearDef_Voltage_L]
    HighVoltage -> Normal : [BatteryVolt <= RearDef_Voltage_H]
    Normal -> HighVoltage [order 2] : [BatteryVolt > RearDef_Voltage_H]
  state Defrost_Management [parallel]
    settings: executionOrder=2
    state Not_Active
      entry:
      RDStatus = 0;
      TdefCounter = 0;
    state Not_Active_IndicatorOn
      entry:
      RDStatus = 2;
      on every(2,tick):TdefCounter = TdefCounter + 1;
      (default) -> (junction 20)
      (junction 20) -> (junction 22) : [in(Load_Shed_Management.Normal) && RDStatus == 2]
      (junction 22) -> (junction 24) : [MaxDefrostSts == 1 && TdefCounter == 0]
      (junction 24) -> (junction 27) [order 2] : [FirstActivation1 == 0]
      (junction 24) -> (junction 26) [order 1] : [FirstActivation1 == 1]
      (junction 27) -> (junction 33) : {FirstActivation2 = 1}
      (junction 26) -> (junction 30) : {FirstActivation2 = FirstActivation1}
      (junction 30) -> (junction 34)
      (junction 33) -> (junction 34)
    state Active
      entry:
      RDStatus = 1;
      on every(2,tick):TdefCounter = TdefCounter + 1;
    (default) -> Not_Active
    Not_Active -> Not_Active_IndicatorOn [order 1] : [RHWindow == 1 || MaxDefrostSts_OffOn == 1 || DefrostRepetiton_Req == 1]
    Not_Active_IndicatorOn -> Not_Active_IndicatorOn [order 3] : [in(Load_Shed_Management.Normal) && DefrostRepetiton_Req == 0]
    Not_Active_IndicatorOn -> Not_Active [order 2] : [in(Load_Shed_Management.Normal) && (RHWindow == 1 || DefrostRepetiton_Req == 1)]
    (junction 40) -> Not_Active : [MaxDefrostSts_OnOff == 1]
    (junction 38) -> (junction 40) [order 1] : [MaxDefrostSts == 1 && TdefCounter == 0]
    Not_Active_IndicatorOn -> (junction 38) [order 4] : [in(Load_Shed_Management.Normal)]
    (junction 38) -> (junction 43) [order 2] : {RDStatus = 2;
        | TdefCounter = TdefCounter + 1}
    (junction 43) -> (junction 45) [order 1] : [FirstActivation1 == 0]
    (junction 49) -> Not_Active : [TdefCounter > Tdef]
    (junction 45) -> (junction 49) : {FirstActivation2 = 1}
    (junction 43) -> (junction 47) [order 2] : {FirstActivation2 = FirstActivation1}
    (junction 47) -> Not_Active : [TdefCounter > Tdef_Second]
    Not_Active -> Not_Active [order 2] : [DefrostRepetiton_Req == 0]
    Not_Active_IndicatorOn -> Active [order 1] : after(Tbatt2,sec) [in(Load_Shed_Management.HighVoltage)]
    Active -> Not_Active_IndicatorOn [order 2] : [in(Load_Shed_Management.Normal) && DefrostRepetiton_Req == 0]
    Active -> Not_Active_IndicatorOn [order 1] : after(Tbatt1,sec) [in(Load_Shed_Management.LowVoltage)]
  data: FirstActivation1 input; RHWindow input; MaxDefrostSts_OnOff input; MaxDefrostSts input; MaxDefrostSts_OffOn input; DefrostRepetiton_Req input; TdefCounter output; RDStatus output; FirstActivation2 output; Tdef parameter; Tdef_Second parameter; RearDef_Voltage_L parameter; RearDef_Voltage_H parameter; Tbatt1 parameter; Tbatt2 parameter double; BatteryVolt input

== stateflow chart Defrost_3/If Action Subsystem/Chart ==
  state Load_Shed_Management [parallel]
    settings: executionOrder=1
    state LowVoltage
    state Normal
    state HighVoltage
    (default) -> LowVoltage
    LowVoltage -> Normal : [BatteryVolt > RearDef_Voltage_L]
    Normal -> LowVoltage [order 1] : [BatteryVolt <= RearDef_Voltage_L]
    HighVoltage -> Normal : [BatteryVolt <= RearDef_Voltage_H]
    Normal -> HighVoltage [order 2] : [BatteryVolt > RearDef_Voltage_H]
  state Defrost_Management [parallel]
    settings: executionOrder=2
    state Active
      entry:
      FirstActivation = 1;
      RDStatus = 1;
      on every(1,tick):TdefCounter = TdefCounter + 1;
    state Not_Active
      entry:
      FirstActivation = 0;
      RDStatus = 0;
      TdefCounter = 0;
    state NotActive_IndicatorOn
      entry:
      RDStatus = 2;
    (default) -> Not_Active
    Not_Active -> (junction 9) : [IgnOff_ToOn == 1]
    (junction 9) -> Active [order 1] : [RemoteStart == 1 && ExternalTemp ~= SNA && ExternalTemp < Temp_am]
    (junction 9) -> Not_Active [order 2]
    Active -> Not_Active [order 2] : [RemoteStart == 0 || ExternalTemp == SNA || ExternalTemp >= Temp_am]
    NotActive_IndicatorOn -> Active : after(Tbatt2,sec)[in(Load_Shed_Management.HighVoltage)]
    Active -> NotActive_IndicatorOn [order 1] : after(Tbatt1,sec)[in(Load_Shed_Management.LowVoltage)]
  data: BatteryVolt input; RemoteStart input; ExternalTemp input; IgnOff_ToOn input; FirstActivation output; RDStatus output; SNA parameter; TdefCounter output; Temp_am parameter; RearDef_Voltage_L parameter; RearDef_Voltage_H parameter; Tbatt1 parameter; Tbatt2 parameter

== stateflow chart Defrost_3/If Action Subsystem3/Chart ==
  state Not_Active
    entry:
    RDStatus = 0;
  (default) -> Not_Active
  data: RDStatus output

== stateflow chart Defrost_3/Subsystem1/Chart ==
  (default) -> (junction 2)
  (junction 2) -> (junction 11) [order 3] : [RDStatus == 2]
  (junction 2) -> (junction 5) [order 1] : [RDStatus == 0]
  (junction 2) -> (junction 4) [order 2] : [RDStatus == 1]
  (junction 11) -> (junction 13) : {R_DefrostCmd = 0;
      | R_DefrostInfo = 0;
      | CANA_RHWLoadSts = 0;
      | CANB_RHWindowSts = 1;}
  (junction 5) -> (junction 8) : {R_DefrostCmd = 0;
      | R_DefrostInfo = 0;
      | CANA_RHWLoadSts = 0;
      | CANB_RHWindowSts = 0;}
  (junction 4) -> (junction 19) : {R_DefrostCmd = 1;
      | R_DefrostInfo = 1;
      | CANA_RHWLoadSts = 1;
      | CANB_RHWindowSts = 1;}
  (junction 8) -> (junction 21)
  (junction 13) -> (junction 21)
  (junction 19) -> (junction 21)
  data: RDStatus input; CANA_RHWLoadSts output; CANB_RHWindowSts output; R_DefrostCmd output; R_DefrostInfo output

== stateflow chart Defrost_3/If Action Subsystem1/Chart ==
  state Load_Shed_Management [parallel]
    settings: executionOrder=1
    state LowVoltage
    state Normal
    state HighVoltage
    (default) -> LowVoltage
    LowVoltage -> Normal : [BatteryVolt > RearDef_Voltage_L]
    Normal -> LowVoltage [order 1] : [BatteryVolt <= RearDef_Voltage_L]
    HighVoltage -> Normal : [BatteryVolt <= RearDef_Voltage_H]
    Normal -> HighVoltage [order 2] : [BatteryVolt > RearDef_Voltage_H]
  state Defrost_Management [parallel]
    settings: executionOrder=2
    state Not_Active
      entry:
      RDStatus = 0;
      TdefCounter = 0;
    state Acitive
      entry:
      RDStatus = 1;
      TdefCounter = 1;
      on every(1,tick):TdefCounter = TdefCounter + 1;
      (default) -> (junction 14)
      (junction 14) -> (junction 16) : [RDStatus == 1]
      (junction 16) -> (junction 18) : [MaxDefrostSts ==1 && TdefCounter == 0]
      (junction 18) -> (junction 27) [order 2] : [FirstActivation == 1]
      (junction 18) -> (junction 23) [order 1] : [FirstActivation == 0]
      (junction 27) -> (junction 29) : {FirstActivation1 = FirstActivation}
      (junction 23) -> (junction 25) : {FirstActivation1 = 1}
      (junction 29) -> (junction 31)
      (junction 25) -> (junction 31)
    state Not_Active_indicatorOn
      entry:
      RDStatus = 2;
      TdefCounter = 0;
    (default) -> Not_Active
    Not_Active -> Acitive : [RHWindow == 1 || MaxDefrostSts_OffOn == 1 || DefrostRepetiton_Req == 1]
    Acitive -> Not_Active [order 2] : [RHWindow == 1 || MaxDefrostSts_OffOn == 1]
    (junction 36) -> Not_Active : [MaxDefrostSts_OnOff == 1]
    (junction 34) -> (junction 36) [order 1] : [MaxDefrostSts ==1 && TdefCounter == 0]
    Acitive -> (junction 34) [order 3]
    (junction 34) -> (junction 46) [order 2] : {RDStatus = 1;
        | TdefCounter = TdefCounter + 1;}
    (junction 42) -> Not_Active : [TdefCounter > Tdef]
    (junction 40) -> (junction 42) : {FirstActivation1 = 1}
    (junction 46) -> (junction 40) [order 1] : [FirstActivation == 0]
    (junction 46) -> (junction 44) [order 2] : {FirstActivation1 = FirstActivation}
    (junction 44) -> Not_Active : [TdefCounter > Tdef_Second]
    Not_Active_indicatorOn -> Not_Active [order 2] : [in(Load_Shed_Management.Normal) && (RHWindow == 1 || DefrostRepetiton_Req == 1)]
    Not_Active_indicatorOn -> Acitive [order 3] : [in(Load_Shed_Management.Normal) && DefrostRepetiton_Req == 0]
    Not_Active_indicatorOn -> Acitive [order 1] : after(Tbatt2,sec)[in(Load_Shed_Management.HighVoltage)]
    Acitive -> Not_Active_indicatorOn [order 1] : after(Tbatt1,sec)[in(Load_Shed_Management.LowVoltage)]
  data: FirstActivation input; RHWindow input; MaxDefrostSts_OffOn input; MaxDefrostSts input; MaxDefrostSts_OnOff input; DefrostRepetiton_Req input; RDStatus output; TdefCounter output; Tdef parameter; Tdef_Second parameter; FirstActivation1 output; Tbatt1 parameter; Tbatt2 parameter; BatteryVolt input; RearDef_Voltage_H parameter; RearDef_Voltage_L parameter
